simulink model "FourModesMerged"  (R2022b)
settings: Solver=FixedStepAuto  StartTime=0.0  StopTime=10.0  FixedStep=1e-3  RelTol=1e-3  EnableMultiTasking=on
undefined symbols (not defined in the file): D0, D1, D10, D11, D12, D13, D2, D3, D4, D5, D6, D7, D8, D9, PTA0, PTA1, PTA2, PTB23, PTB9, PTC16, PTC17, PTC2, PTC3, PTC4, PTD0, PTD1, PTD2, PTD3
libraries: frdmk64flib x16
settings Model: ExtModeTrigDuration=5  Creator=16475  LastModifiedBy=kaano
settings OptimizationCC: EnhancedBackFolding=on  PassReuseOutputArgsAs=Individual arguments  ZeroExternalMemoryAtStartup=off  ZeroInternalMemoryAtStartup=off  MaxStackSize=64  OptimizeBlockOrder=speed  DifferentSizesBufferReuse=on  OptimizationCustomize=off  EfficientTunableParamExpr=on
settings DebuggingCC: ParameterTunabilityLossMsg=error
settings HardwareCC: ProdBitPerPointer=32  ProdBitPerSizeT=32  ProdBitPerPtrDiffT=32  ProdLargestAtomicInteger=Long  ProdLargestAtomicFloat=Double  ProdWordSize=32  ProdHWDeviceType=ARM Compatible->ARM Cortex
settings SFSimCC: MATLABDynamicMemAlloc=off
settings RTWCC: Description=Embedded Coder  SystemTargetFile=ert.tlc  HardwareBoard=NXP FRDM-K64F  TLCOptions="-aInlineSetEventsForThisBaseRateFcn=TLC_FALSE -aSuppressMultiTaskScheduler=TLC_FALSE  -aRateBasedStepFcn=0"  TemplateMakefile=ert_default_tmf  Toolchain=GNU Tools for ARM Embedded Processors
settings CodeAppCC: ForceParamTrailComments=on  IgnoreCustomStorageClasses=off  OperatorAnnotations=on  SimulinkDataObjDesc=on  SFDataObjDesc=on  InsertBlockDesc=on
settings ERTTargetCC: ExtModeTransport=4  ExtModeMexFile=sendToCommService

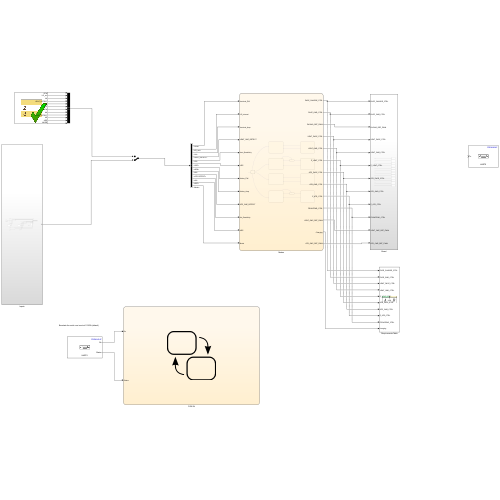
[thumbnail: Simulink's stored preview of the top-level diagram]
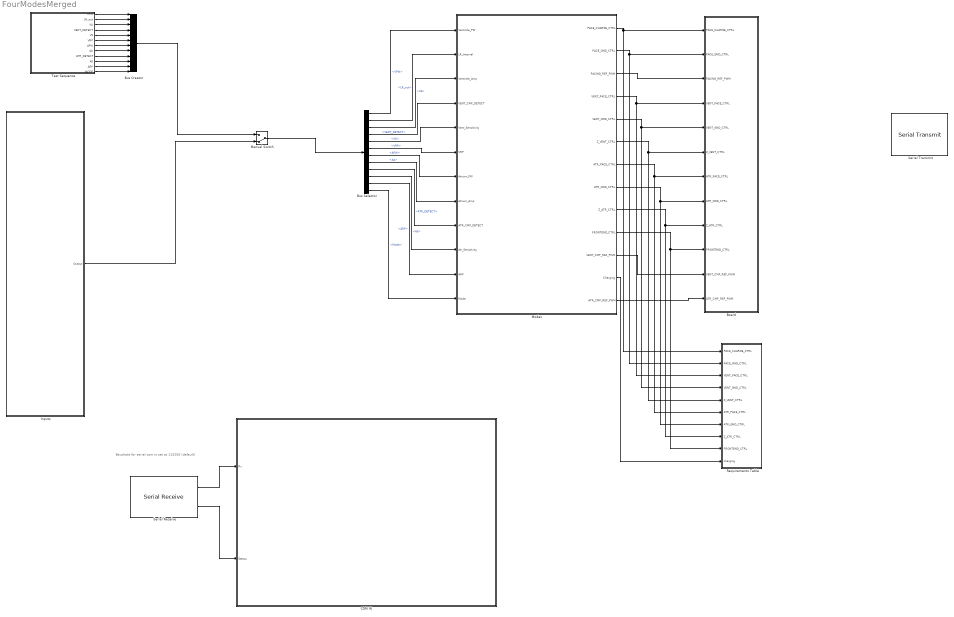
== system FourModesMerged ==
  note: Baudrate for serial com is set at 115200 (default)
  Board : Subsystem
  Bus Creator : BusCreator  Inputs=12
  Bus Selector : BusSelector  OutputSignals=VPW,LR_out,VA,VENT_DETECT,VS,VRP,APW,AA,ATR_DETECT,AS,ARP,Mode
  COM IN : Stateflow chart  TreatAsAtomicUnit=on
  Inputs : Subsystem
  Manual Switch : ManualSwitch  CurrentSetting=0
  Modes : Stateflow chart  TreatAsAtomicUnit=on
      settings: PortSchema="{\"entries\":[{\"content\":{\"sides\":[{\"content\":{\"connectorIds\":[\"In1\",\"In2\",\"In3\",\"In4\",\"In5\",\"In6\",\"In7\",\"In8\",\"In9\",\"In10\",\"In11\",\"In12\"]},\"type\":\"ConnectorPlacement.EquallySpacedRectSide\",\"uuid\":\"a3e94f58-3093-42a5-91db-f56c9d127bee\"},{\"content\":{\"connectorIds\":[\"Out1\",\"Out2\",\"Out3\",\"Out5\",\"Out4\",\"Out7\",\"Out6\",\"Out8\",\"Out9\",\"Out10\",\"Out11\",\"Out12\",\"Out13\"],\"side\":\"RIGHT\"},\"type\":\"ConnectorPlacement.EquallySpacedRectSide\",\"uuid\":\"289ad049-9840-4721-af22-1385d5696f7c\"},{\"content\":{\"connectorIds\":[],\"side\":\"TOP\"},\"type\":\"ConnectorPlacement.EquallySpacedRectSide\",\"uuid\":\"4602f2ad-cb91-4c7a-9db6-6571445db01f\"}]},\"type\":\"ConnectorPlacement.EquallySpacedConnector\",\"uuid\":\"bfd50937-4990-4c1b-ba87-ff4dc7d3240f\"}],\"packageUris\":[\"http://schema.mathworks.com/mf0/Connector/R2020b\"],\"version\":\"1.0\"}"
  Requirements Table : Requirements Table  TreatAsAtomicUnit=on
  Serial Receive : frdmk64flib/Serial Receive  SCIModule=0  Baudrate=uint32(9600)  Parity=None  StopBits=1  HardwareFlowControl=None  ByteOrder=LittleEndian  DataType=uint8  DataLength=10  BlockingMode=off  OutputStatus=on  SampleTime=-1
  Serial Transmit : frdmk64flib/Serial Transmit  SCIModule=0  Baudrate=uint32(9600)  Parity=None  StopBits=1  HardwareFlowControl=None  ByteOrder=LittleEndian  BlockingMode=on  OutputStatus=off
  Test Sequence : Test Sequence  TreatAsAtomicUnit=on
  wires:
  Modes/11(VENT_CMP_REF_PWM) -> Board/11(VENT_CMP_REF_PWM)
  Modes/1(PACE_CHARGE_CTRL) -> Requirements Table/1(PACE_CHARGE_CTRL), Board/1(PACE_CHARGE_CTRL)
  Modes/2(PACE_GND_CTRL) -> Requirements Table/2(PACE_GND_CTRL), Board/2(PACE_GND_CTRL)
  Modes/3(PACING_REF_PWM) -> Board/3(PACING_REF_PWM)
  Modes/5(VENT_PACE_CTRL) -> Requirements Table/3(VENT_PACE_CTRL), Board/4(VENT_PACE_CTRL)
  Modes/4(VENT_GND_CTRL) -> Requirements Table/4(VENT_GND_CTRL), Board/5(VENT_GND_CTRL)
  Modes/7(Z_VENT_CTRL) -> Requirements Table/5(Z_VENT_CTRL), Board/6(Z_VENT_CTRL)
  Modes/6(ATR_PACE_CTRL) -> Requirements Table/6(ATR_PACE_CTRL), Board/7(ATR_PACE_CTRL)
  Modes/8(ATR_GND_CTRL) -> Requirements Table/7(ATR_GND_CTRL), Board/8(ATR_GND_CTRL)
  Modes/9(Z_ATR_CTRL) -> Requirements Table/8(Z_ATR_CTRL), Board/9(Z_ATR_CTRL)
  Modes/10(FRONTEND_CTRL) -> Requirements Table/9(FRONTEND_CTRL), Board/10(FRONTEND_CTRL)
  Modes/12(Charging) -> Requirements Table/10(charging)
  Modes/13(ATR_CMP_REF_PWM) -> Board/12(ATR_CMP_REF_PWM)
  Bus Selector/1 -> Modes/1(Ventricle_PW)  "<VPW>"
  Bus Selector/2 -> Modes/2(LR_Interval)  "<LR_out>"
  Bus Selector/3 -> Modes/3(Ventricle_Amp)  "<VA>"
  Bus Selector/4 -> Modes/4(VENT_CMP_DETECT)  "<VENT_DETECT>"
  Bus Selector/5 -> Modes/5(Vent_Sensitivity)  "<VS>"
  Bus Selector/6 -> Modes/6(VRP)  "<VRP>"
  Bus Selector/7 -> Modes/7(Atrium_PW)  "<APW>"
  Bus Selector/8 -> Modes/8(Atrium_Amp)  "<AA>"
  Bus Selector/9 -> Modes/9(ATR_CMP_DETECT)  "<ATR_DETECT>"
  Bus Selector/10 -> Modes/10(Atr_Sensitivity)  "<AS>"
  Bus Selector/11 -> Modes/11(ARP)  "<ARP>"
  Bus Selector/12 -> Modes/12(Mode)  "<Mode>"
  Test Sequence/1(VPW) -> Bus Creator/1
  Test Sequence/2(LR_out) -> Bus Creator/2
  Test Sequence/3(VA) -> Bus Creator/3
  Test Sequence/4(VENT_DETECT) -> Bus Creator/4
  Test Sequence/5(VS) -> Bus Creator/5
  Test Sequence/6(VRP) -> Bus Creator/6
  Test Sequence/7(APW) -> Bus Creator/7
  Test Sequence/8(AA) -> Bus Creator/8
  Test Sequence/9(ATR_DETECT) -> Bus Creator/9
  Test Sequence/10(AS) -> Bus Creator/10
  Test Sequence/11(ARP) -> Bus Creator/11
  Test Sequence/12(MODE) -> Bus Creator/12
  Bus Creator/1 -> Manual Switch/1
  Inputs/1(Output) -> Manual Switch/2
  Manual Switch/1 -> Bus Selector/1
  Serial Receive/1 -> COM IN/1(Rx)
  Serial Receive/2 -> COM IN/2(Status)

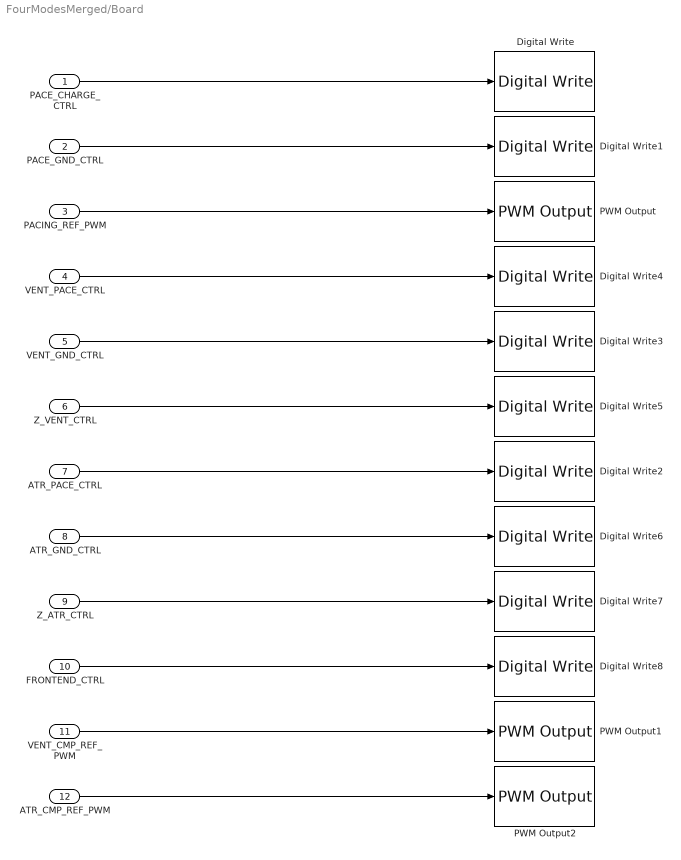
== system FourModesMerged/Board ==
  PACE_CHARGE_CTRL : Inport
  PACE_GND_CTRL : Inport  Port=2
  PACING_REF_PWM : Inport  Port=3
  VENT_PACE_CTRL : Inport  Port=4
  VENT_GND_CTRL : Inport  Port=5
  Z_VENT_CTRL : Inport  Port=6
  ATR_PACE_CTRL : Inport  Port=7
  ATR_GND_CTRL : Inport  Port=8
  Z_ATR_CTRL : Inport  Port=9
  FRONTEND_CTRL : Inport  Port=10
  VENT_CMP_REF_PWM : Inport  Port=11
  ATR_CMP_REF_PWM : Inport  Port=12
  Digital Write : frdmk64flib/Digital Write  Whichpin=PTB9 (D2)
  Digital Write1 : frdmk64flib/Digital Write  Whichpin=PTD0 (D10)
  Digital Write2 : frdmk64flib/Digital Write  Whichpin=PTA0 (D8)
  Digital Write3 : frdmk64flib/Digital Write  Whichpin=PTD3 (D12)
  Digital Write4 : frdmk64flib/Digital Write  Whichpin=PTC4 (D9)
  Digital Write5 : frdmk64flib/Digital Write  Whichpin=PTC3 (D7)
  Digital Write6 : frdmk64flib/Digital Write  Whichpin=PTD2 (D11)
  Digital Write7 : frdmk64flib/Digital Write  Whichpin=PTB23 (D4)
  Digital Write8 : frdmk64flib/Digital Write  Whichpin=PTD1 (D13)
  PWM Output : frdmk64flib/PWM Output  Whichpin=PTA2 (D5)  InitialFrequency=2000  InitialDutyCycle=0
  PWM Output1 : frdmk64flib/PWM Output  Whichpin=PTA1 (D3)  InitialFrequency=2000  InitialDutyCycle=0
  PWM Output2 : frdmk64flib/PWM Output  Whichpin=PTC2 (D6)  InitialFrequency=2000  InitialDutyCycle=0
  wires:
  Z_VENT_CTRL/1 -> Digital Write5/1
  VENT_GND_CTRL/1 -> Digital Write3/1
  PACE_CHARGE_CTRL/1 -> Digital Write/1
  PACE_GND_CTRL/1 -> Digital Write1/1
  VENT_PACE_CTRL/1 -> Digital Write4/1
  ATR_GND_CTRL/1 -> Digital Write6/1
  ATR_PACE_CTRL/1 -> Digital Write2/1
  PACING_REF_PWM/1 -> PWM Output/1
  Z_ATR_CTRL/1 -> Digital Write7/1
  FRONTEND_CTRL/1 -> Digital Write8/1
  VENT_CMP_REF_PWM/1 -> PWM Output1/1
  ATR_CMP_REF_PWM/1 -> PWM Output2/1

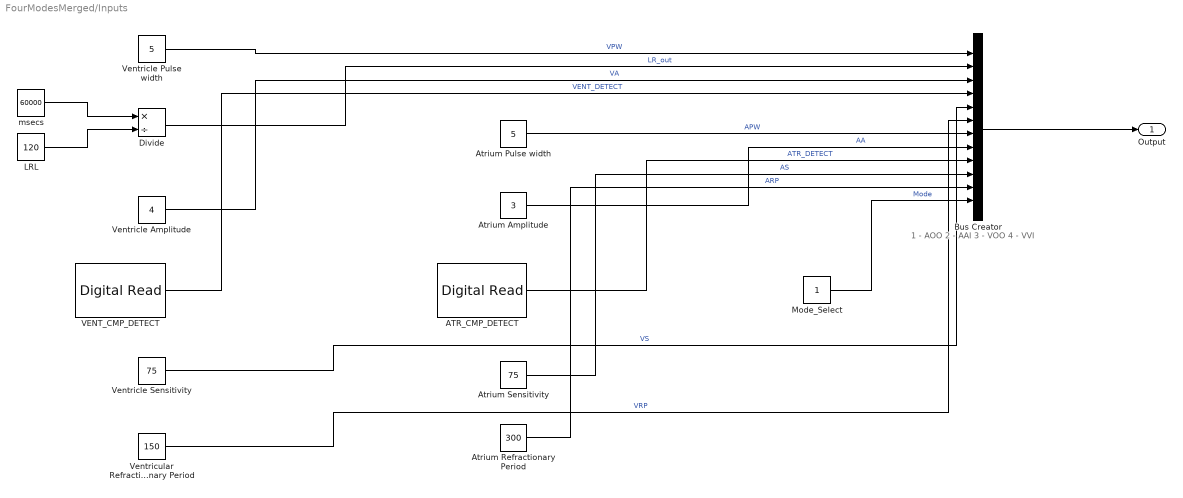
== system FourModesMerged/Inputs ==
  note: 1 - AOO
      | 2 - AAI
      | 3 - VOO
      | 4 - VVI
  ATR_CMP_DETECT : frdmk64flib/Digital Read  Whichpin=PTC16 (D0)  SampleTime=-1
  Atrium Amplitude : Constant  Value=3
  Atrium Pulse width : Constant  Value=5
  Atrium Refractionary Period : Constant  Value=300
  Atrium Sensitivity : Constant  Value=75
  Bus Creator : BusCreator  Inputs=12
  Divide : Product  Inputs=*/
  LRL : Constant  Value=120
  Mode_Select : Constant
  VENT_CMP_DETECT : frdmk64flib/Digital Read  Whichpin=PTC17 (D1)  SampleTime=-1
  Ventricle Amplitude : Constant  Value=4
  Ventricle Pulse width : Constant  Value=5
  Ventricle Sensitivity : Constant  Value=75
  Ventricular Refractionary Period : Constant  Value=150
  msecs : Constant  Value=60000
  Output : Outport
  wires:
  msecs/1 -> Divide/1
  LRL/1 -> Divide/2
  Bus Creator/1 -> Output/1
  Ventricle Pulse width/1 -> Bus Creator/1  "VPW"
  Divide/1 -> Bus Creator/2  "LR_out"
  Ventricle Amplitude/1 -> Bus Creator/3  "VA"
  VENT_CMP_DETECT/1 -> Bus Creator/4  "VENT_DETECT"
  Ventricle Sensitivity/1 -> Bus Creator/5  "VS"
  Ventricular Refractionary Period/1 -> Bus Creator/6  "VRP"
  Atrium Pulse width/1 -> Bus Creator/7  "APW"
  Atrium Amplitude/1 -> Bus Creator/8  "AA"
  ATR_CMP_DETECT/1 -> Bus Creator/9  "ATR_DETECT"
  Atrium Sensitivity/1 -> Bus Creator/10  "AS"
  Atrium Refractionary Period/1 -> Bus Creator/11  "ARP"
  Mode_Select/1 -> Bus Creator/12  "Mode"

== stateflow chart FourModesMerged/Modes ==
  state Charging_AOO
    entry:
    ATR_PACE_CTRL = false;
    VENT_PACE_CTRL = false;
    PACING_REF_PWM = ((Atrium_Amp/5)*100);
    PACE_CHARGE_CTRL = true;
    PACE_GND_CTRL = true;
    Z_ATR_CTRL = false;
    Z_VENT_CTRL = false;
    ATR_GND_CTRL = true;
    VENT_GND_CTRL = false;
    Charging = true;
  state Discharging_AOO
    entry:
    PACE_CHARGE_CTRL = false;
    PACE_GND_CTRL = true;
    ATR_PACE_CTRL = true;
    VENT_PACE_CTRL = false;
    Z_ATR_CTRL = false;
    Z_VENT_CTRL = false;
    ATR_GND_CTRL = false;
    VENT_GND_CTRL = false;
    Charging = false;
  state Charging_AAI
    entry:
    ATR_PACE_CTRL = false;
    VENT_PACE_CTRL = false;
    PACING_REF_PWM = ((Atrium_Amp/5)*100);
    PACE_CHARGE_CTRL = true;
    PACE_GND_CTRL = true;
    Z_ATR_CTRL = false;
    Z_VENT_CTRL = false;
    ATR_GND_CTRL = true;
    VENT_GND_CTRL = false;
    FRONTEND_CTRL = true;
    ATR_CMP_REF_PWM = Atr_Sensitivity;
    Charging = true;
  state Discharging_AAI
    entry:
    PACE_CHARGE_CTRL = false;
    PACE_GND_CTRL = true;
    ATR_PACE_CTRL = true;
    VENT_PACE_CTRL = false;
    Z_ATR_CTRL = false;
    Z_VENT_CTRL = false;
    ATR_GND_CTRL = false;
    VENT_GND_CTRL = false;
    FRONTEND_CTRL = false;
    Charging = false;
  state Check_State_AAI
  state Init
  state Charging_VOO
    entry:
    ATR_PACE_CTRL = false;
    VENT_PACE_CTRL = false;
    PACING_REF_PWM = ((Ventricle_Amp/5)*100);
    PACE_CHARGE_CTRL = true;
    PACE_GND_CTRL = true;
    Z_ATR_CTRL = false;
    Z_VENT_CTRL = false;
    ATR_GND_CTRL = false;
    VENT_GND_CTRL = true;
    Charging = true;
  state Discharging_VOO
    entry:
    PACE_CHARGE_CTRL = false;
    PACE_GND_CTRL = true;
    ATR_PACE_CTRL = false;
    VENT_PACE_CTRL = true;
    Z_ATR_CTRL = false;
    Z_VENT_CTRL = false;
    ATR_GND_CTRL = false;
    VENT_GND_CTRL = false;
    Charging = false;
  state Charging_Sensing_VVI
    entry:
    ATR_PACE_CTRL = false;
    VENT_PACE_CTRL = false;
    PACING_REF_PWM = ((Ventricle_Amp/5)*100);
    PACE_CHARGE_CTRL = true;
    PACE_GND_CTRL = true;
    Z_ATR_CTRL = false;
    Z_VENT_CTRL = false;
    ATR_GND_CTRL = false;
    VENT_GND_CTRL = true;
    FRONTEND_CTRL = true;
    VENT_CMP_REF_PWM = Vent_Sensitivity;
    Charging = true;
  state Discharging_VVI
    entry:
    PACE_CHARGE_CTRL = false;
    PACE_GND_CTRL = true;
    ATR_PACE_CTRL = false;
    VENT_PACE_CTRL = true;
    Z_ATR_CTRL = false;
    Z_VENT_CTRL = false;
    ATR_GND_CTRL = false;
    VENT_GND_CTRL = false;
    FRONTEND_CTRL = false;
    Charging = false;
  state Check_State_VVI
  Charging_AOO -> Discharging_AOO : [after(LR_Interval - Atrium_PW,msec)]
  Init -> Charging_AOO [order 1] : [Mode == 1]
  Discharging_AOO -> Charging_AOO : [after(Atrium_PW,msec)]
  Check_State_AAI -> Charging_AAI [order 1] : [ATR_CMP_DETECT == true]
  Charging_AAI -> Check_State_AAI : [after(ARP,msec)]
  Check_State_AAI -> Discharging_AAI [order 2] : [after(LR_Interval - ARP,msec)]
  Init -> Charging_AAI [order 2] : [Mode == 2]
  Discharging_AAI -> Charging_AAI : [after(Atrium_PW,msec)]
  (default) -> Init
  Init -> Charging_VOO [order 3] : [Mode == 3]
  Init -> Charging_Sensing_VVI [order 4] : [Mode == 4]
  Charging_VOO -> Discharging_VOO : [after(LR_Interval - Ventricle_PW,msec)]
  Discharging_VOO -> Charging_VOO : [after(Ventricle_PW,msec)]
  Check_State_VVI -> Charging_Sensing_VVI [order 1] : [VENT_CMP_DETECT == true]
  Check_State_VVI -> Discharging_VVI [order 2] : [after(LR_Interval - VRP,msec)]
  Charging_Sensing_VVI -> Check_State_VVI : [after(VRP,msec)]
  Discharging_VVI -> Charging_Sensing_VVI : [after(Ventricle_PW,msec)]
  data: Ventricle_PW input double; LR_Interval input double; PACE_CHARGE_CTRL output boolean; PACE_GND_CTRL output boolean; PACING_REF_PWM output double; VENT_GND_CTRL output boolean; VENT_PACE_CTRL output boolean; ATR_PACE_CTRL output boolean; Z_VENT_CTRL output boolean; Ventricle_Amp input double; ATR_GND_CTRL output boolean; Z_ATR_CTRL output boolean; VENT_CMP_DETECT input boolean; FRONTEND_CTRL output boolean; VENT_CMP_REF_PWM output double; Vent_Sensitivity input double; VRP input double; Charging output; Atrium_PW input; Atrium_Amp input; ATR_CMP_DETECT input; Atr_Sensitivity input; ARP input; Mode input; ATR_CMP_REF_PWM output

== stateflow chart FourModesMerged/Requirements Table ==
  (default) -> (junction 1073742521)
  (junction 1073742521) -> (junction 1073742522) : {
      | % SF_REQ_REV_07
      | }
  (junction 1073742522) -> (junction 1073742524) : {
      | % HEADER_ASSIGNMENTS
      |
      | }
  (junction 1073742524) -> (junction 1073742526) : {
      | % START_A_4
      | }
  (junction 1073742526) -> (junction 1073742528) : {
      | }
  (junction 1073742528) -> (junction 1073742530)
  (junction 1073742530) -> (junction 1073742532) : {
      | }
  (junction 1073742532) -> (junction 1073742534) : {
      | % END_A_4
      | }
  (junction 1073742534) -> (junction 1073742536) : {
      | % START_R_1
      | }
  (junction 1073742536) -> (junction 1073742538) : {
      | }
  (junction 1073742538) -> (junction 1073742540)
  (junction 1073742540) -> (junction 1073742542) [order 1] : [(prev(charging) == false)]
  (junction 1073742540) -> (junction 1073742548) [order 2]
  (junction 1073742542) -> (junction 1073742544) : {
      | reqtable_postcondition((((PACE_CHARGE_CTRL) == (true))) && (((PACE_GND_CTRL) == (true))) && (((VENT_PACE_CTRL) == (false))) && (((VENT_GND_CTRL) == (true))) && (((Z_VENT_CTRL) == (false))) && (((ATR_PACE_CTRL) == (false))) && (((ATR_GND_CTRL) == (false))) && (((Z_ATR_CTRL) == (false))) && (((FRONTEND_CTRL) == (true))) && (((charging) == (true))), 'R:1');
      |
      |
      | }
  (junction 1073742544) -> (junction 1073742546) : {
      | }
  (junction 1073742546) -> (junction 1073742548)
  (junction 1073742548) -> (junction 1073742550)
  (junction 1073742550) -> (junction 1073742552) : {
      | % END_R_1
      | }
  (junction 1073742552) -> (junction 1073742554) : {
      | % START_R_7
      | }
  (junction 1073742554) -> (junction 1073742556) : {
      | }
  (junction 1073742556) -> (junction 1073742558)
  (junction 1073742558) -> (junction 1073742560) [order 1] : [(prev(charging) == true)]
  (junction 1073742558) -> (junction 1073742566) [order 2]
  (junction 1073742560) -> (junction 1073742562) : {
      | reqtable_postcondition((((PACE_CHARGE_CTRL) == (false))) && (((PACE_GND_CTRL) == (true))) && (((VENT_PACE_CTRL) == (true))) && (((VENT_GND_CTRL) == (false))) && (((Z_VENT_CTRL) == (false))) && (((ATR_PACE_CTRL) == (false))) && (((ATR_GND_CTRL) == (false))) && (((Z_ATR_CTRL) == (false))) && (((FRONTEND_CTRL) == (false))) && (((charging) == (false))), 'R:2');
      |
      |
      | }
  (junction 1073742562) -> (junction 1073742564) : {
      | }
  (junction 1073742564) -> (junction 1073742566)
  (junction 1073742566) -> (junction 1073742568)
  (junction 1073742568) -> (junction 1073742570) : {
      | % END_R_7
      | }
  data: PACE_CHARGE_CTRL input boolean; PACE_GND_CTRL input boolean; VENT_PACE_CTRL input boolean; VENT_GND_CTRL input boolean; Z_VENT_CTRL input boolean; ATR_PACE_CTRL input boolean; ATR_GND_CTRL input boolean; Z_ATR_CTRL input boolean; FRONTEND_CTRL input boolean; charging input boolean

== stateflow chart FourModesMerged/COM IN ==
  data: Rx input; Status input

== stateflow chart FourModesMerged/Test Sequence ==
  state step_1
    Msecs = 60000;
    LRL = 120;
    VPW =5;
    LR_out = Msecs/LRL;
    VA=4;
    VS=75;
    VRP=150;
    APW=5;
    AA=3;
    AS=75;
    ARP=300
    state step_1_1
      ATR_DETECT = 0;
      VENT_DETECT=0;
      settings: description=AOO
    state step_1_2
      ATR_DETECT=1;
      VENT_DETECT=0;
      settings: description=AAI
    state step_1_3
      VENT_DETECT=0;
      ATR_DETECT=0;
      settings: description=VOO
    state step_1_4
      VENT_DETECT=1;
      ATR_DETECT=0;
      settings: description=VVI
    (default) -> step_1_1
  state step_2
  (default) -> step_1
  step_1 -> step_2
  data: VPW output; LR_out output; VA output; VENT_DETECT output; VS output; VRP output; APW output; AA output; ATR_DETECT output; AS output; ARP output; MODE output
